simulink model "RocketLander_version2"  (R2023a)
settings: Solver=VariableStepAuto  StartTime=0.0  StopTime=10  MaxStep=1E-3  RelTol=1e-3
model workspace (MAT data in the model file):
  Gimbal_Angle = 0
  gravity = 1
  mass = 1.2
libraries: simulink x2
settings Model: Creator=lukea  LastModifiedBy=lukea

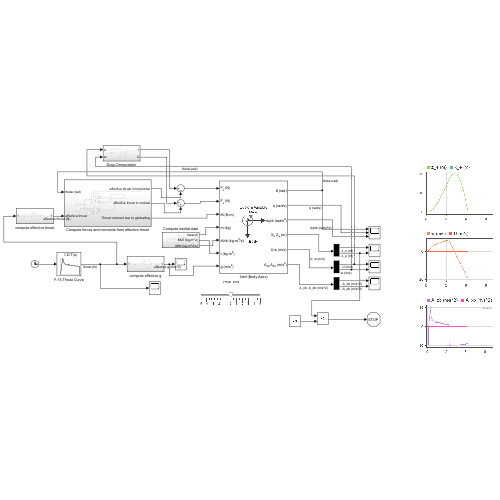
[thumbnail: Simulink's stored preview of the top-level diagram]
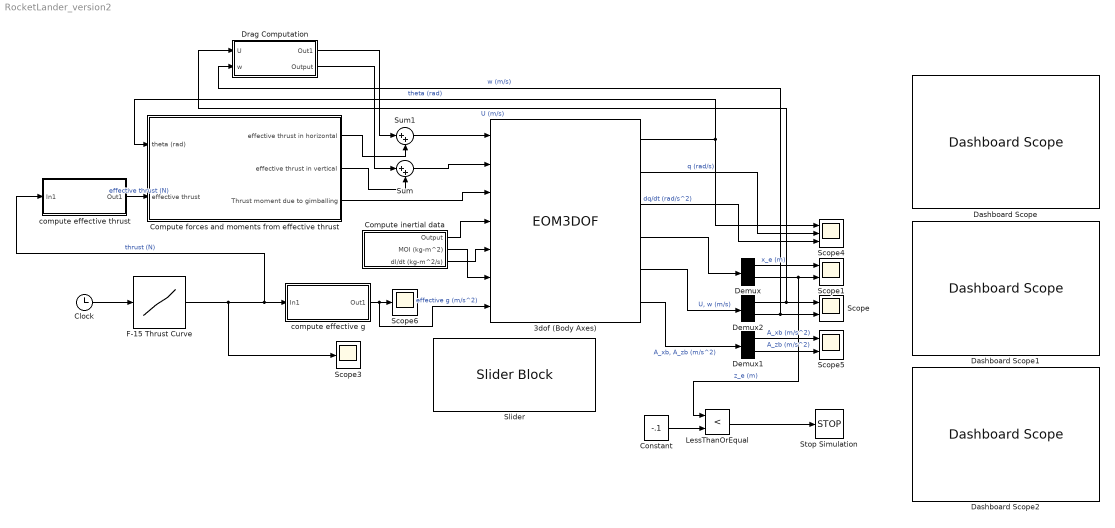
== system RocketLander_version2 ==
  3dof (Body Axes) : EOM3DOF  mtype=Custom Variable  v_ini=0  mass=mass  Iyy=1.5  g_in=External
  Clock : Clock
  Compute forces and moments from effective thrust : Subsystem
  Compute inertial data : Subsystem
  Constant : Constant  Value=-.1
  Dashboard Scope : DashboardScope
  Dashboard Scope1 : DashboardScope
  Dashboard Scope2 : DashboardScope
  Demux : Demux  Outputs=2
  Demux1 : Demux  Outputs=2
  Demux2 : Demux  Outputs=2
  Drag Computation : Subsystem
  F-15 Thrust Curve : Lookup_n-D  NumberOfTableDimensions=1  BreakpointsForDimension1=[0;0.148;0.228;0.294;0.353;0.382;0.419;0.477;0.52;0.593;0.688;0.855;1.037;1.205;1.423;1.452;1.503;1.736;1.955;2.21;2.494;2.763;3.12;3.382;3.404;3.418;3.45]  Table=[0;7.638;12.253;16.391;20.21;22.756;25.26;23.074;20.845;19.093;17.5;16.225;15.427;14.948;14.627;15.741;14.785;14.623;14.303;14.141;13.819;13.338;13.334;13.013;9.352;4.895;0]  ExtrapMethod=Clip  UseLastTableValue=on  InternalRulePriority=Speed  RndMeth=Simplest
  LessThanOrEqual : RelationalOperator  Operator=<  OutDataTypeStr=boolean  RndMeth=Simplest  InputSameDT=off
  Scope : Scope  NumInputPorts=2
  Scope1 : Scope  NumInputPorts=2
  Scope3 : Scope
  Scope4 : Scope  NumInputPorts=3
  Scope5 : Scope  NumInputPorts=2
  Scope6 : Scope
  Slider : SliderBlock  ScaleMin=-5  ScaleMax=5  TickInterval=1
  Stop Simulation : Stop
  Sum : Sum  Inputs=|++
  Sum1 : Sum  Inputs=|++
  compute effective g : Subsystem
  compute effective thrust : Subsystem
  wires:
  Clock/1 -> F-15 Thrust Curve/1
  F-15 Thrust Curve/1 -> Scope3/1, compute effective thrust/1(In1), compute effective g/1(In1)  "thrust (N)"
  3dof (Body Axes)/1 -> Compute forces and moments from effective thrust/1(theta (rad)), Scope4/1  "theta (rad)"
  3dof (Body Axes)/4 -> Demux/1
  3dof (Body Axes)/6 -> Demux1/1  "A_xb, A_zb (m/s^2)"
  Demux/1 -> Scope1/1  "x_e (m)"
  3dof (Body Axes)/2 -> Scope4/2  "q (rad/s)"
  3dof (Body Axes)/3 -> Scope4/3  "dq/dt (rad/s^2)"
  3dof (Body Axes)/5 -> Demux2/1  "U, w (m/s)"
  Demux2/1 -> Drag Computation/1(U), Scope/1  "U (m/s)"
  Demux2/2 -> Drag Computation/2(w), Scope/2  "w (m/s)"
  Demux1/1 -> Scope5/1  "A_xb (m/s^2)"
  Demux1/2 -> Scope5/2  "A_zb (m/s^2)"
  compute effective g/1(Out1) -> 3dof (Body Axes)/7, Scope6/1  "effective g (m/s^2)"
  compute effective thrust/1(Out1) -> Compute forces and moments from effective thrust/2(effective thrust)  "effective thrust (N)"
  Compute forces and moments from effective thrust/2(effective thrust in vertical) -> Sum/2
  Compute forces and moments from effective thrust/3(Thrust moment due to gimballing) -> 3dof (Body Axes)/3
  Demux/2 -> LessThanOrEqual/1, Scope1/2  "z_e (m)"
  Sum/1 -> 3dof (Body Axes)/2
  Sum1/1 -> 3dof (Body Axes)/1
  Compute forces and moments from effective thrust/1(effective thrust in horizontal) -> Sum1/2
  Drag Computation/1(Out1) -> Sum1/1
  Drag Computation/2(Output) -> Sum/1
  LessThanOrEqual/1 -> Stop Simulation/1
  Constant/1 -> LessThanOrEqual/2
  Compute inertial data/1(Output) -> 3dof (Body Axes)/4
  Compute inertial data/2(MOI (kg-m^2)) -> 3dof (Body Axes)/6
  Compute inertial data/3(dI/dt (kg-m^2/s)) -> 3dof (Body Axes)/5

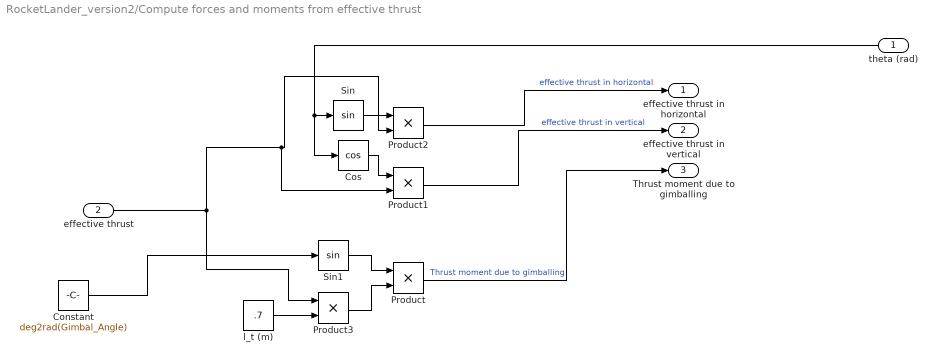
== system RocketLander_version2/Compute forces and moments from effective thrust ==
  theta (rad) : Inport
  effective thrust : Inport  Port=2
  Constant : Constant  Value=deg2rad(Gimbal_Angle)
  Cos : Trigonometry  Operator=cos
  Product{,1..3} (4 alike) : Product
  Sin : Trigonometry
  Sin1 : Trigonometry
  l_t (m) : Constant  Value=.7
  effective thrust in horizontal : Outport
  effective thrust in vertical : Outport  Port=2
  Thrust moment due to gimballing : Outport  Port=3
  wires:
  Cos/1 -> Product1/1
  effective thrust/1 -> Product1/2, Product2/2, Product3/1
  theta (rad)/1 -> Sin/1, Cos/1
  Sin/1 -> Product2/1
  Sin1/1 -> Product/1
  Product/1 -> Thrust moment due to gimballing/1  "Thrust moment due to gimballing"
  Product3/1 -> Product/2
  l_t (m)/1 -> Product3/2
  Product1/1 -> effective thrust in vertical/1  "effective thrust in vertical"
  Product2/1 -> effective thrust in horizontal/1  "effective thrust in horizontal"
  Constant/1 -> Sin1/1

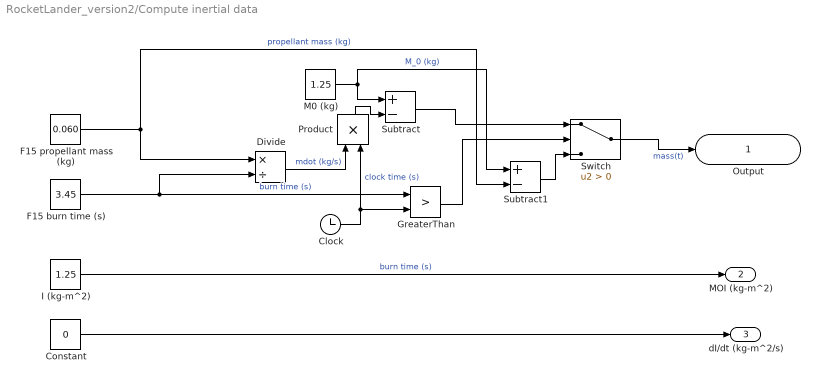
== system RocketLander_version2/Compute inertial data ==
  Clock : Clock
  Constant : Constant  Value=0
  Divide : Product  Inputs=*/
  F15 burn time (s) : Constant  Value=3.45
  F15 propellant mass (kg) : Constant  Value=0.060
  GreaterThan : RelationalOperator  Operator=>  OutDataTypeStr=boolean  RndMeth=Simplest  InputSameDT=off
  I (kg-m^2) : Constant  Value=1.25
  M0 (kg) : Constant  Value=1.25
  Product : Product
  Subtract : Sum  Inputs=+-
  Subtract1 : Sum  Inputs=+-
  Switch : Switch  Criteria=u2 > Threshold  SaturateOnIntegerOverflow=off  InputSameDT=off
  Output : Outport
  MOI (kg-m^2) : Outport  Port=2
  dI/dt (kg-m^2/s) : Outport  Port=3
  wires:
  Switch/1 -> Output/1  "mass(t)"
  Clock/1 -> GreaterThan/2, Product/2  "clock time (s)"
  F15 burn time (s)/1 -> Divide/2, GreaterThan/1  "burn time (s)"
  GreaterThan/1 -> Switch/2
  Subtract/1 -> Switch/1
  M0 (kg)/1 -> Subtract1/1, Subtract/1  "M_0 (kg)"
  F15 propellant mass (kg)/1 -> Divide/1, Subtract1/2  "propellant mass (kg)"
  Divide/1 -> Product/1  "mdot (kg/s)"
  Product/1 -> Subtract/2
  Subtract1/1 -> Switch/3
  I (kg-m^2)/1 -> MOI (kg-m^2)/1  "burn time (s)"
  Constant/1 -> dI/dt (kg-m^2/s)/1

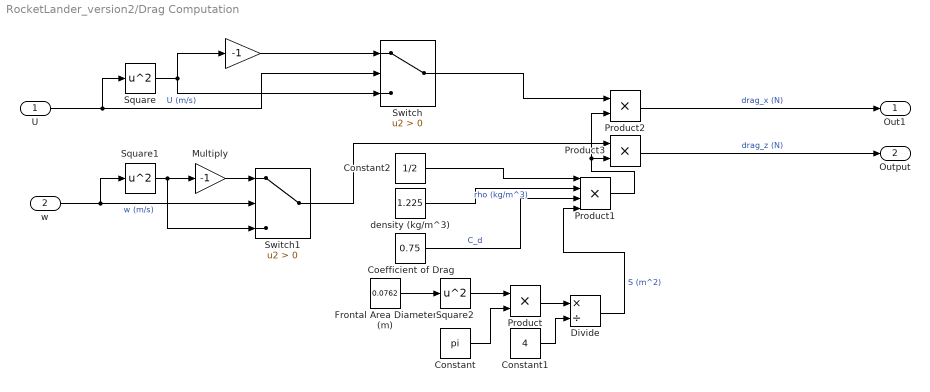
== system RocketLander_version2/Drag Computation ==
  U : Inport
  w : Inport  Port=2
  " " : Gain  Gain=-1
  Coefficient of Drag : Constant  Value=0.75
  Constant : Constant  Value=pi
  Constant1 : Constant  Value=4
  Constant2 : Constant  Value=1/2
  Divide : Product  Inputs=*/
  Frontal Area Diameter (m) : Constant  Value=0.0762
  Multiply : Gain  Gain=-1
  Product : Product
  Product1 : Product  Inputs=4
  Product2 : Product
  Product3 : Product
  Square : Math  Operator=square
  Square1 : Math  Operator=square
  Square2 : Math  Operator=square
  Switch : Switch  Criteria=u2 > Threshold  SaturateOnIntegerOverflow=off  InputSameDT=off
  Switch1 : Switch  Criteria=u2 > Threshold  SaturateOnIntegerOverflow=off  InputSameDT=off
  density (kg/m^3) : Constant  Value=1.225
  Out1 : Outport
  Output : Outport  Port=2
  wires:
  w/1 -> Switch1/2, Square1/1  "w (m/s)"
  Frontal Area Diameter (m)/1 -> Square2/1
  Square2/1 -> Product/1
  Constant/1 -> Product/2
  Product/1 -> Divide/1
  Constant1/1 -> Divide/2
  Divide/1 -> Product1/4  "S (m^2)"
  Coefficient of Drag/1 -> Product1/3  "C_d"
  density (kg/m^3)/1 -> Product1/2  "rho (kg/m^3)"
  Square/1 -> Switch/3, " "/1
  Product1/1 -> Product2/2, Product3/2
  Product2/1 -> Out1/1  "drag_x (N)"
  Product3/1 -> Output/1  "drag_z (N)"
  Constant2/1 -> Product1/1
  Switch/1 -> Product2/1
  U/1 -> Square/1, Switch/2  "U (m/s)"
  " "/1 -> Switch/1
  Square1/1 -> Switch1/3, Multiply/1
  Multiply/1 -> Switch1/1
  Switch1/1 -> Product3/1

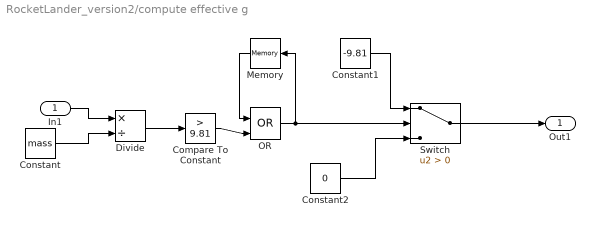
== system RocketLander_version2/compute effective g ==
  In1 : Inport
  Compare To Constant : simulink/Logic and Bit Operations/Compare To Constant  relop=>  const=9.81  OutDataTypeStr=boolean
  Constant : Constant  Value=mass
  Constant1 : Constant  Value=-9.81
  Constant2 : Constant  Value=0
  Divide : Product  Inputs=*/
  Memory : Memory
  OR : Logic  Operator=OR  IconShape=distinctive  AllPortsSameDT=off  OutDataTypeStr=boolean
  Switch : Switch  Criteria=u2 > Threshold  SaturateOnIntegerOverflow=off  InputSameDT=off
  Out1 : Outport
  wires:
  In1/1 -> Divide/1
  Constant/1 -> Divide/2
  Divide/1 -> Compare To Constant/1
  Compare To Constant/1 -> OR/2
  OR/1 -> Switch/2, Memory/1
  Memory/1 -> OR/1
  Constant1/1 -> Switch/1
  Constant2/1 -> Switch/3
  Switch/1 -> Out1/1

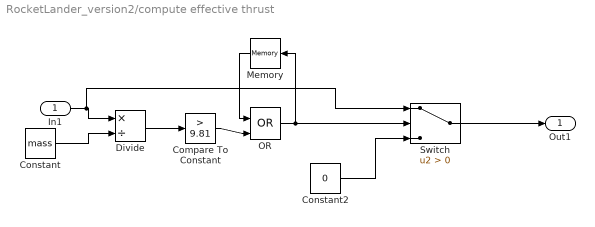
== system RocketLander_version2/compute effective thrust ==
  In1 : Inport
  Compare To Constant : simulink/Logic and Bit Operations/Compare To Constant  relop=>  const=9.81  OutDataTypeStr=boolean
  Constant : Constant  Value=mass
  Constant2 : Constant  Value=0
  Divide : Product  Inputs=*/
  Memory : Memory
  OR : Logic  Operator=OR  IconShape=distinctive  AllPortsSameDT=off  OutDataTypeStr=boolean
  Switch : Switch  Criteria=u2 > Threshold  SaturateOnIntegerOverflow=off  InputSameDT=off
  Out1 : Outport
  wires:
  Constant/1 -> Divide/2
  Divide/1 -> Compare To Constant/1
  Compare To Constant/1 -> OR/2
  OR/1 -> Switch/2, Memory/1
  Memory/1 -> OR/1
  In1/1 -> Switch/1, Divide/1
  Constant2/1 -> Switch/3
  Switch/1 -> Out1/1
